simulink model "twoLinkManipulator"  (R2020a)
settings: Solver=ode45  StartTime=0.0  StopTime=20  MaxStep=0.01  RelTol=1e-3
undefined symbols (not defined in the file): DESIRED_TRAJECTORY_IS_FIXED, dq_max, dq_min, k1, k2, k3, q_des_amp, q_des_bias, q_des_freq, q_des_phase, q_max, q_min
libraries: sm_lib x9, nesl_utility x9
settings Model: Creator=bpc  LastModifiedBy=bpc
settings ExplorerConfigSet: InternalSimMechanicsExplorerSettings="<ExplorerConfiguration><canonicalview>aerospace</canonicalview><AnimationSetting><BasePlaybackSpeed>1.0</BasePlaybackSpeed><PlaybackSpeedFactor>1.0</PlaybackSpeedFactor></AnimationSetting><TilePanel><TileInfo><Tiles Columns=\"1\" Count=\"1\" Rows=\"1\"><Column Weight=\"1\"/><Row Weight=\"1\"/><Tile Height=\"1\" Width=\"1\" X=\"0\" Y=\"0\"/></Tiles></TileInfo><SceneInfo><SceneViewer><BGColor><R>0.800000011920928955</R><G>0.800000011920928955</G><B>0.800000011920928955</B></BGColor><Camera><DoPerspective>off</DoPerspective><Position><X>0.880734530182891495</X><Y>-0.069313660265544183</Y><Z>1.00000000000000044</Z></Position><Center><X>0.880734530182891495</X><Y>-0.069313660265544183</Y><Z>4.44089209850062616e-16</Z></Center><Up><X>0</X><Y>1</Y><Z>-0</Z></Up><ViewLimDist>1</ViewLimDist><YLim>0.716863440183610257</YLim><XLim>1.28420727523043032</XLim></Camera></SceneViewer></SceneInfo></TilePanel><MechEditorPanel><Cameras/><GfxPanelCameraMap/><VideoCreator><PlaybackSpeedRatio>1.0</PlaybackSpeedRatio><FrameRate>30</FrameRate><VideoFormat>Motion JPEG AVI</VideoFormat><FrameSize>auto</FrameSize></VideoCreator></MechEditorPanel></ExplorerConfiguration>"

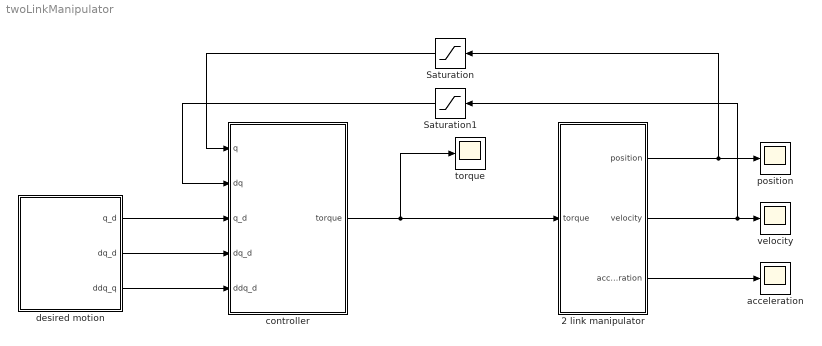
== system twoLinkManipulator ==
  2 link manipulator : Subsystem
  Saturation : Saturate  UpperLimit=q_max-0.001  LowerLimit=q_min+0.001
  Saturation1 : Saturate  UpperLimit=dq_max-0.001  LowerLimit=dq_min+0.001
  acceleration : Scope
  controller : Subsystem
  desired motion : Subsystem
  position : Scope
  torque : Scope
  velocity : Scope
  wires:
  2 link manipulator/1(position) -> Saturation/1, position/1
  2 link manipulator/2(velocity) -> Saturation1/1, velocity/1
  2 link manipulator/3(acceleration) -> acceleration/1
  controller/1(torque) -> 2 link manipulator/1(torque), torque/1
  desired motion/1(q_d) -> controller/3(q_d)
  desired motion/2(dq_d) -> controller/4(dq_d)
  desired motion/3(ddq_q) -> controller/5(ddq_d)
  Saturation/1 -> controller/1(q)
  Saturation1/1 -> controller/2(dq)

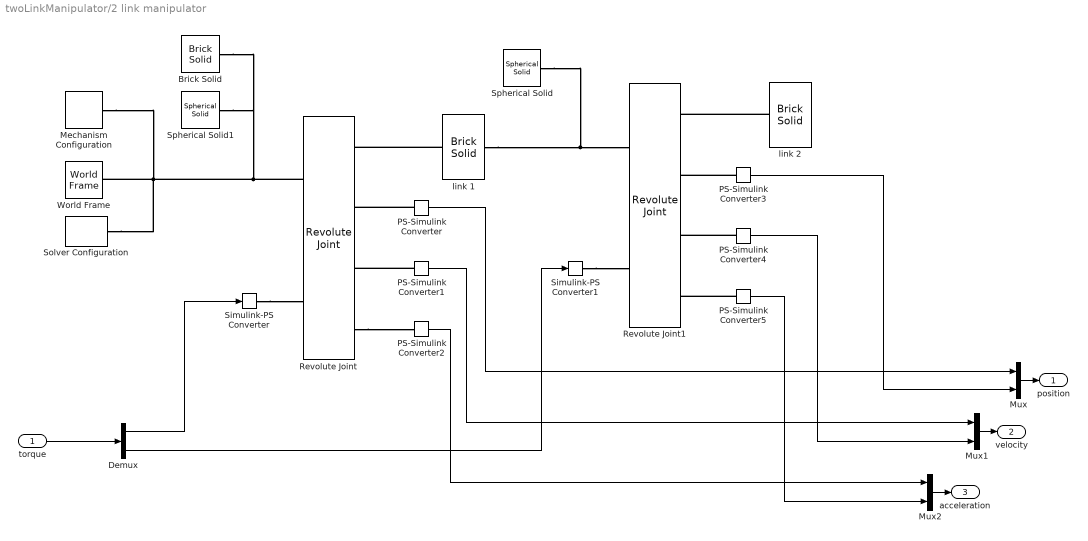
== system twoLinkManipulator/2 link manipulator ==
  torque : Inport
  Brick Solid : sm_lib/Body Elements/Brick Solid  GraphicAmbientColor=[0.15 0.15 0.15 1.0]  BasedOnType=Density  BrickDimensions=[0.2 0.5 0.5]  BrickDimensionUnits=m  CenterOfMass=[0 0 0]  CenterOfMassUnits=m  GraphicDiffuseColor=[0.5 0.5 0.5]  Density=1000  DensityUnits=kg/m^3  DoExposeReferenceFrame=off  GraphicEmissiveColor=[0.0 0.0 0.0 1.0]  ExportEntireGeometry=off  SerializedFrames=<Frames><Frame><Id>Frame1</Id><Value><Name>F1</Name><Origin><Source>GeometricFeature</Source><FeatureName>+x surface</FeatureName></Origin><PrimaryAxis><DefinedDirection>+Z</DefinedDirection><Source>ReferenceFrame</Source><SourceDirection>+Z</SourceDirection><FeatureName></FeatureName></PrimaryAxis><SecondaryAxis><DefinedDirection>+X</DefinedDirection><Source>ReferenceFrame</Source><SourceDirection>+X</SourceDirection><FeatureName></FeatureName></SecondaryAxis></Value></Frame></Frames>  MarkerShape=Sphere  MarkerSize=10  GraphicType=FromGeometry  InertiaType=PointMass  Mass=0.0  MassUnits=kg  MomentsOfInertia=[1 1 1]  MomentsOfInertiaUnits=kg*m^2  GraphicOpacity=1.0  ProductsOfInertia=[0 0 0]  ProductsOfInertiaUnits=kg*m^2  GraphicShininess=75  GraphicSpecularColor=[0.5 0.5 0.5 1.0]  GraphicVisPropType=SimpleVisualProperties
  Demux : Demux  Outputs=2
  Mechanism Configuration : sm_lib/Utilities/Mechanism Configuration  UniformGravity=Constant  GravityVector=[0 -9.80665 0]  GravityUnits=m/s^2  LinearizationDelta=0.001
  Mux : Mux  Inputs=2
  Mux1 : Mux  Inputs=2
  Mux2 : Mux  Inputs=2
  PS-Simulink Converter{,1..5} (6 alike) : nesl_utility/PS-Simulink Converter  PhysicalDomain=network_engine_domain  SubClassName=ps_output  LeftPortType=input  RightPortType=output  PseudoPeriodic=off  Frequencies=[]  Unit=inherit  AffineConversion=off
  Revolute Joint : sm_lib/Joints/Revolute Joint  JointMode=Normal  SenseConstraintForce=off  SenseConstraintForceX=off  SenseConstraintForceY=off  SenseConstraintForceZ=off  SenseConstraintTorque=off  SenseConstraintTorqueX=off  SenseConstraintTorqueY=off  SenseConstraintTorqueZ=off  SenseTotalForce=off  SenseTotalForceX=off  SenseTotalForceY=off  SenseTotalForceZ=off  SenseTotalTorque=off  SenseTotalTorqueX=off  SenseTotalTorqueY=off  SenseTotalTorqueZ=off  CompositeWrenchDir=FollowerOnBase  CompositeWrenchFrame=BaseFrame  EquilibriumPosition=0  EquilibriumPositionUnits=deg  SpringStiffness=0  SpringStiffnessUnits=N*m/deg  DampingCoefficient=0  DampingCoefficientUnits=N*m/(deg/s)  TorqueActuationMode=InputTorque  MotionActuationMode=ComputedMotion  SensePosition=on  SenseVelocity=on  SenseAcceleration=on  SenseTorqueForce=off  SenseLowerLimitTorqueForce=off  SenseUpperLimitTorqueForce=off  LowerLimitSpecify=on  LowerLimitBound=-90  LowerLimitBoundUnits=deg  LowerLimitStiffness=1e4  LowerLimitStiffnessUnits=N*m/deg  LowerLimitDamping=10  LowerLimitDampingUnits=N*m/(deg/s)  LowerLimitTransitionRegionWidth=0.1  LowerLimitTransitionRegionWidthUnits=deg  UpperLimitSpecify=on  UpperLimitBound=90  UpperLimitBoundUnits=deg  UpperLimitStiffness=1e4  UpperLimitStiffnessUnits=N*m/deg  UpperLimitDamping=10  UpperLimitDampingUnits=N*m/(deg/s)  UpperLimitTransitionRegionWidth=0.1  UpperLimitTransitionRegionWidthUnits=deg  PositionTargetSpecify=off  PositionTargetPriority=High  PositionTargetValue=pi/10  PositionTargetValueUnits=rad  VelocityTargetSpecify=off  VelocityTargetPriority=High  VelocityTargetValue=0  VelocityTargetValueUnits=deg/s
  Revolute Joint1 : sm_lib/Joints/Revolute Joint  JointMode=Normal  SenseConstraintForce=off  SenseConstraintForceX=off  SenseConstraintForceY=off  SenseConstraintForceZ=off  SenseConstraintTorque=off  SenseConstraintTorqueX=off  SenseConstraintTorqueY=off  SenseConstraintTorqueZ=off  SenseTotalForce=off  SenseTotalForceX=off  SenseTotalForceY=off  SenseTotalForceZ=off  SenseTotalTorque=off  SenseTotalTorqueX=off  SenseTotalTorqueY=off  SenseTotalTorqueZ=off  CompositeWrenchDir=FollowerOnBase  CompositeWrenchFrame=BaseFrame  EquilibriumPosition=0  EquilibriumPositionUnits=deg  SpringStiffness=0  SpringStiffnessUnits=N*m/deg  DampingCoefficient=0  DampingCoefficientUnits=N*m/(deg/s)  TorqueActuationMode=InputTorque  MotionActuationMode=ComputedMotion  SensePosition=on  SenseVelocity=on  SenseAcceleration=on  SenseTorqueForce=off  SenseLowerLimitTorqueForce=off  SenseUpperLimitTorqueForce=off  LowerLimitSpecify=on  LowerLimitBound=-90  LowerLimitBoundUnits=deg  LowerLimitStiffness=1e4  LowerLimitStiffnessUnits=N*m/deg  LowerLimitDamping=10  LowerLimitDampingUnits=N*m/(deg/s)  LowerLimitTransitionRegionWidth=0.1  LowerLimitTransitionRegionWidthUnits=deg  UpperLimitSpecify=on  UpperLimitBound=90  UpperLimitBoundUnits=deg  UpperLimitStiffness=1e4  UpperLimitStiffnessUnits=N*m/deg  UpperLimitDamping=10  UpperLimitDampingUnits=N*m/(deg/s)  UpperLimitTransitionRegionWidth=0.1  UpperLimitTransitionRegionWidthUnits=deg  PositionTargetSpecify=off  PositionTargetPriority=High  PositionTargetValue=0  PositionTargetValueUnits=deg  VelocityTargetSpecify=off  VelocityTargetPriority=High  VelocityTargetValue=0  VelocityTargetValueUnits=deg/s
  Simulink-PS Converter : nesl_utility/Simulink-PS Converter  PhysicalDomain=network_engine_domain  SubClassName=ps_input  LeftPortType=input  RightPortType=output  PseudoPeriodic=off  Frequencies=[]  NoiseDistribution=none  NoiseParameters=[]  Unit=1  AffineConversion=off  FilteringAndDerivatives=provide  SimscapeFilterOrder=1  InputFilterTimeConstant=0.001  UdotUserProvided=0
  Simulink-PS Converter1 : nesl_utility/Simulink-PS Converter  PhysicalDomain=network_engine_domain  SubClassName=ps_input  LeftPortType=input  RightPortType=output  PseudoPeriodic=off  Frequencies=[]  NoiseDistribution=none  NoiseParameters=[]  Unit=1  AffineConversion=off  FilteringAndDerivatives=provide  SimscapeFilterOrder=1  InputFilterTimeConstant=0.001  UdotUserProvided=0
  Solver Configuration : nesl_utility/Solver Configuration  PhysicalDomain=network_engine_domain  SubClassName=solver  LeftPortType=input  RightPortType=generic  Tones=[]  Harmonics=[]  SimulateNoise=off  Profile=off  UseLocalSampling=off  EnableSwitchedLinearOptims=on  FrequencyDomain=off  UseCCode=off  RelTol=0.001  AbsTol=1e-06  MinStep=1e-09  ToWorkspace=off  RevertToSquareIcSolve=off  NumHomotopyIterations=100  PhasorMode=off  PhasorModeNumHarmonics=1  DoDC=off  ResidualTolerance=1e-09  UseLocalSolver=off  LocalSolverChoice=NE_BACKWARD_EULER_ADVANCER  LocalSolverSampleTime=0.001  DoFixedCost=off  MaxNonlinIter=3  MaxModeIter=2  LinearAlgebra=auto  EquationFormulation=NE_TIME_EF  DelaysMemoryBudget=1024  AutomaticFiltering=on  FilteringTimeConstant=0.001  PartitionStorageMethod=AS_NEEDED  PartitionMemoryBudget=1024  PartitionMethod=ROBUST
  Spherical Solid : sm_lib/Body Elements/Spherical Solid  GraphicAmbientColor=[0.15 0.15 0.15 1.0]  BasedOnType=Density  CenterOfMass=[0 0 0]  CenterOfMassUnits=m  GraphicDiffuseColor=[1.0 0.6 0.2]  Density=1000  DensityUnits=kg/m^3  DoExposeReferenceFrame=on  GraphicEmissiveColor=[0.0 0.0 0.0 1.0]  ExportEntireGeometry=off  SerializedExposedGeometries=<ExposedGeometries/>  SerializedFrames=<Frames/>  MarkerShape=Sphere  MarkerSize=10  GraphicType=FromGeometry  InertiaType=PointMass  Mass=0.0  MassUnits=kg  MomentsOfInertia=[1 1 1]  MomentsOfInertiaUnits=kg*m^2  GraphicOpacity=1.0  ProductsOfInertia=[0 0 0]  ProductsOfInertiaUnits=kg*m^2  GraphicShininess=75  GraphicSpecularColor=[0.5 0.5 0.5 1.0]  SphereRadius=0.02  SphereRadiusUnits=m  GraphicVisPropType=SimpleVisualProperties
  Spherical Solid1 : sm_lib/Body Elements/Spherical Solid  GraphicAmbientColor=[0.15 0.15 0.15 1.0]  BasedOnType=Density  CenterOfMass=[0 0 0]  CenterOfMassUnits=m  GraphicDiffuseColor=[1.0 0.6 0.2]  Density=1000  DensityUnits=kg/m^3  DoExposeReferenceFrame=on  GraphicEmissiveColor=[0.0 0.0 0.0 1.0]  ExportEntireGeometry=off  SerializedExposedGeometries=<ExposedGeometries/>  SerializedFrames=<Frames/>  MarkerShape=Sphere  MarkerSize=10  GraphicType=FromGeometry  InertiaType=PointMass  Mass=0.0  MassUnits=kg  MomentsOfInertia=[1 1 1]  MomentsOfInertiaUnits=kg*m^2  GraphicOpacity=1.0  ProductsOfInertia=[0 0 0]  ProductsOfInertiaUnits=kg*m^2  GraphicShininess=75  GraphicSpecularColor=[0.5 0.5 0.5 1.0]  SphereRadius=0.02  SphereRadiusUnits=m  GraphicVisPropType=SimpleVisualProperties
  World Frame : sm_lib/Frames and Transforms/World Frame
  link 1 : sm_lib/Body Elements/Brick Solid  GraphicAmbientColor=[0.15 0.15 0.15 1.0]  BasedOnType=Density  BrickDimensions=[0.5 0.015 0.015]  BrickDimensionUnits=m  CenterOfMass=[0.25 0.0075 0.0075]  CenterOfMassUnits=m  GraphicDiffuseColor=[0.0 0.0 1.0]  Density=1000  DensityUnits=kg/m^3  DoExposeReferenceFrame=off  GraphicEmissiveColor=[0.0 0.0 0.0 1.0]  ExportEntireGeometry=off  SerializedFrames=<Frames><Frame><Id>Frame1</Id><Value><Name>F1</Name><Origin><Source>GeometricFeature</Source><FeatureName>-x surface</FeatureName></Origin><PrimaryAxis><DefinedDirection>+Z</DefinedDirection><Source>ReferenceFrame</Source><SourceDirection>+Z</SourceDirection><FeatureName></FeatureName></PrimaryAxis><SecondaryAxis><DefinedDirection>+X</DefinedDirection><Source>ReferenceFrame</Source><SourceDirection>+X</SourceDirection><FeatureName></FeatureName></SecondaryAxis></Value></Frame><Frame><Id>Frame2</Id><Value><Name>F2</Name><Origin><Source>GeometricFeature</Source><FeatureName>+x surface</FeatureName></Origin><PrimaryAxis><DefinedDirection>+Z</DefinedDirection><Source>ReferenceFrame</Source><SourceDirection>+Z</SourceDirection><FeatureName></FeatureName></PrimaryAxis><SecondaryAxis><DefinedDirection>+X</DefinedDirection><Source>ReferenceFrame</Source><SourceDirection>+X</SourceDirection><FeatureName></FeatureName></SecondaryAxis></Value></Frame></Frames>  MarkerShape=Sphere  MarkerSize=10  GraphicType=FromGeometry  InertiaType=PointMass  Mass=2  MassUnits=kg  MomentsOfInertia=[0 0.0417 0]  MomentsOfInertiaUnits=kg*m^2  GraphicOpacity=1.0  ProductsOfInertia=[0 0 0]  ProductsOfInertiaUnits=kg*m^2  GraphicShininess=75  GraphicSpecularColor=[0.5 0.5 0.5 1.0]  GraphicVisPropType=SimpleVisualProperties
  link 2 : sm_lib/Body Elements/Brick Solid  GraphicAmbientColor=[0.15 0.15 0.15 1.0]  BasedOnType=Density  BrickDimensions=[0.35 0.015 0.015]  BrickDimensionUnits=m  CenterOfMass=[0.175 0.0075 0.0075]  CenterOfMassUnits=m  GraphicDiffuseColor=[0.0 1.0 0.2]  Density=1000  DensityUnits=kg/m^3  DoExposeReferenceFrame=off  GraphicEmissiveColor=[0.0 0.0 0.0 1.0]  ExportEntireGeometry=off  SerializedFrames=<Frames><Frame><Id>Frame1</Id><Value><Name>F1</Name><Origin><Source>GeometricFeature</Source><FeatureName>-x surface</FeatureName></Origin><PrimaryAxis><DefinedDirection>+Z</DefinedDirection><Source>ReferenceFrame</Source><SourceDirection>+Z</SourceDirection><FeatureName></FeatureName></PrimaryAxis><SecondaryAxis><DefinedDirection>+X</DefinedDirection><Source>ReferenceFrame</Source><SourceDirection>+X</SourceDirection><FeatureName></FeatureName></SecondaryAxis></Value></Frame></Frames>  MarkerShape=Sphere  MarkerSize=10  GraphicType=FromGeometry  InertiaType=PointMass  Mass=1.5  MassUnits=kg  MomentsOfInertia=[0 0.0153 0]  MomentsOfInertiaUnits=kg*m^2  GraphicOpacity=1.0  ProductsOfInertia=[0 0 0]  ProductsOfInertiaUnits=kg*m^2  GraphicShininess=75  GraphicSpecularColor=[0.5 0.5 0.5 1.0]  GraphicVisPropType=SimpleVisualProperties
  position : Outport
  velocity : Outport  Port=2
  acceleration : Outport  Port=3
  wires:
  PS-Simulink Converter/1 -> Mux/1
  PS-Simulink Converter5/1 -> Mux2/2
  PS-Simulink Converter3/1 -> Mux/2
  PS-Simulink Converter4/1 -> Mux1/2
  PS-Simulink Converter1/1 -> Mux1/1
  PS-Simulink Converter2/1 -> Mux2/1
  Mux2/1 -> acceleration/1
  Mux1/1 -> velocity/1
  Mux/1 -> position/1
  torque/1 -> Demux/1
  Demux/1 -> Simulink-PS Converter/1
  Demux/2 -> Simulink-PS Converter1/1
  connections:
  PS-Simulink Converter5/LConn1 -- Revolute Joint1/RConn4
  PS-Simulink Converter4/LConn1 -- Revolute Joint1/RConn3
  link 1/RConn1 -- Spherical Solid/RConn1 -- Revolute Joint1/LConn1
  PS-Simulink Converter3/LConn1 -- Revolute Joint1/RConn2
  Revolute Joint/LConn1 -- Brick Solid/LConn1 -- Spherical Solid1/RConn1 -- Solver Configuration/RConn1 -- Mechanism Configuration/RConn1 -- World Frame/RConn1
  PS-Simulink Converter/LConn1 -- Revolute Joint/RConn2
  link 1/LConn1 -- Revolute Joint/RConn1
  PS-Simulink Converter1/LConn1 -- Revolute Joint/RConn3
  Revolute Joint/RConn4 -- PS-Simulink Converter2/LConn1
  link 2/LConn1 -- Revolute Joint1/RConn1
  Simulink-PS Converter/RConn1 -- Revolute Joint/LConn2
  Simulink-PS Converter1/RConn1 -- Revolute Joint1/LConn2

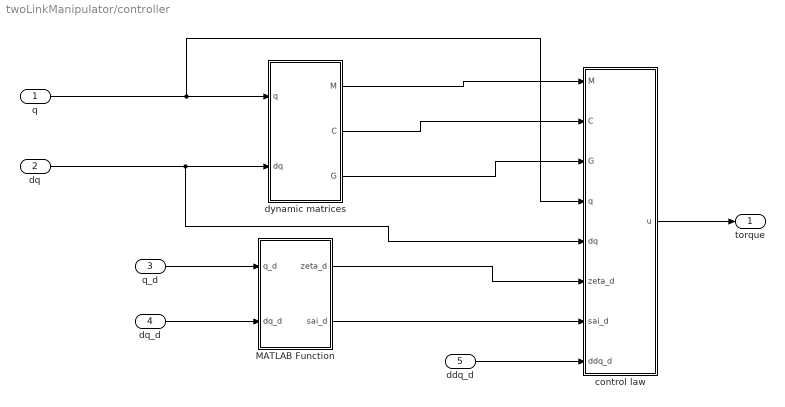
== system twoLinkManipulator/controller ==
  q : Inport
  dq : Inport  Port=2
  q_d : Inport  Port=3
  dq_d : Inport  Port=4
  ddq_d : Inport  Port=5
  MATLAB Function : MATLAB Function  TreatAsAtomicUnit=on
  control law : MATLAB Function  TreatAsAtomicUnit=on
  dynamic matrices : MATLAB Function  TreatAsAtomicUnit=on
  torque : Outport
  wires:
  q/1 -> control law/4(q), dynamic matrices/1(q)
  dq/1 -> control law/5(dq), dynamic matrices/2(dq)
  dynamic matrices/1(M) -> control law/1(M)
  dynamic matrices/2(C) -> control law/2(C)
  dynamic matrices/3(G) -> control law/3(G)
  ddq_d/1 -> control law/8(ddq_d)
  control law/1(u) -> torque/1
  MATLAB Function/1(zeta_d) -> control law/6(zeta_d)
  MATLAB Function/2(sai_d) -> control law/7(sai_d)
  q_d/1 -> MATLAB Function/1(q_d)
  dq_d/1 -> MATLAB Function/2(dq_d)

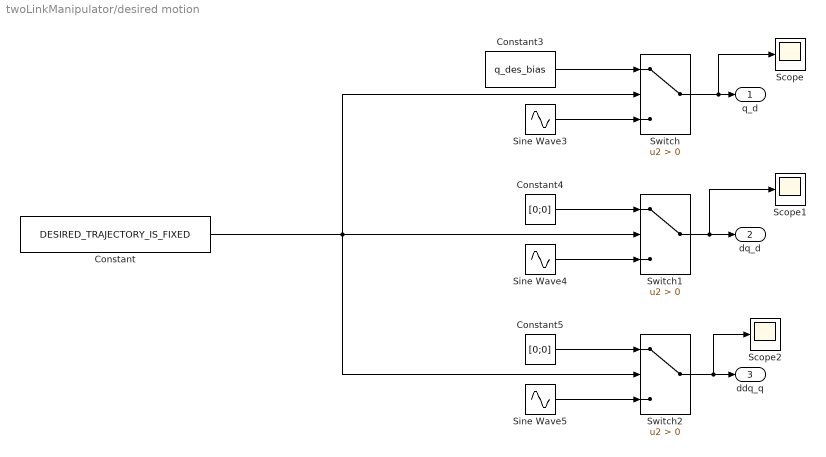
== system twoLinkManipulator/desired motion ==
  Constant : Constant  Value=DESIRED_TRAJECTORY_IS_FIXED
  Constant3 : Constant  Value=q_des_bias
  Constant4 : Constant  Value=[0;0]
  Constant5 : Constant  Value=[0;0]
  Scope : Scope
  Scope1 : Scope
  Scope2 : Scope
  Sine Wave3 : Sin  Amplitude=q_des_amp  Bias=q_des_bias  Frequency=q_des_freq  Phase=q_des_phase  SampleTime=0
  Sine Wave4 : Sin  Amplitude=q_des_amp .* q_des_freq  Bias=[0;0]  Frequency=q_des_freq  Phase=q_des_phase+pi/2  SampleTime=0
  Sine Wave5 : Sin  Amplitude=-q_des_amp .* (q_des_freq .^ 2)  Bias=[0;0]  Frequency=q_des_freq  Phase=q_des_phase  SampleTime=0
  Switch : Switch  Criteria=u2 > Threshold
  Switch1 : Switch  Criteria=u2 > Threshold
  Switch2 : Switch  Criteria=u2 > Threshold
  q_d : Outport
  dq_d : Outport  Port=2
  ddq_q : Outport  Port=3
  wires:
  Switch/1 -> Scope/1, q_d/1
  Switch1/1 -> Scope1/1, dq_d/1
  Switch2/1 -> Scope2/1, ddq_q/1
  Constant/1 -> Switch1/2, Switch2/2, Switch/2
  Constant3/1 -> Switch/1
  Sine Wave3/1 -> Switch/3
  Sine Wave4/1 -> Switch1/3
  Constant4/1 -> Switch1/1
  Constant5/1 -> Switch2/1
  Sine Wave5/1 -> Switch2/3

== matlab function twoLinkManipulator/controller/control law ==
  data: M input; C input; G input; q input; u output; dq input; zeta_d input; sai_d input; ddq_d input; q_min parameter; q_max parameter; dq_min parameter; dq_max parameter; k1 parameter; k2 parameter; k3 parameter
function u = fcn(M,C,G,q,dq,zeta_d,sai_d,ddq_d, q_min, q_max, dq_min, dq_max, k1, k2, k3)

%%%%%%%%%%%%%%%%%%%%%%%%%%%%%%%%%%%%%%%%%%%%%%%%%%%%%%%%%%%%%%%%%%%%%%%%%

q_avg = (q_max+q_min)/2;
dq_avg = (dq_max+dq_min)/2;

delta_q = diag((q_max-q_min)/2);
delta_dq = diag((dq_max-dq_min)/2);

%%%%%%%%%%%%%%%%%%%%%%%%%%%%%%%%%%%%%%%%%%%%%%%%%%%%%%%%%%%%%%%%%%%%%%%%%

zeta = atanh(delta_q\(q-q_avg));
sai = atanh(delta_dq\(dq-dq_avg));

%%%%%%%%%%%%%%%%%%%%%%%%%%%%%%%%%%%%%%%%%%%%%%%%%%%%%%%%%%%%%%%%%%%%%%%%%

J_zeta = delta_q*(eye(2)-diag(tanh(zeta))^2);
J_zeta_d = delta_q*(eye(2)-diag(tanh(zeta_d))^2);

J_sai = delta_dq*(eye(2)-diag(tanh(sai))^2);
J_sai_d = delta_dq*(eye(2)-diag(tanh(sai_d))^2);

%%%%%%%%%%%%%%%%%%%%%%%%%%%%%%%%%%%%%%%%%%%%%%%%%%%%%%%%%%%%%%%%%%%%%%%%%

dzeta = J_zeta\(dq_avg + delta_dq*tanh(sai));
dzeta_d = J_zeta_d\(dq_avg + delta_dq*tanh(sai_d));

dJ_zeta = -2*diag(tanh(zeta))*J_zeta*diag(dzeta);
dJ_zeta_d = -2*diag(tanh(zeta_d))*J_zeta_d*diag(dzeta_d);

dsai_d = J_sai_d\ddq_d;

%%%%%%%%%%%%%%%%%%%%%%%%%%%%%%%%%%%%%%%%%%%%%%%%%%%%%%%%%%%%%%%%%%%%%%%%%

p = 15;

tanh_bsai_r = delta_dq\(J_zeta/J_zeta_d*(dq_avg+delta_dq*tanh(sai_d)) - dq_avg);
sai_r =  atanh(tanh_bsai_r./(1+abs(tanh_bsai_r).^p).^(1/p));

J_sai_r = delta_dq*(eye(2)-diag(tanh(sai_r))^2);

dsai_r = J_sai_r\(dJ_zeta/J_zeta_d*(dq_avg+delta_dq*tanh(sai_d)) ...
    -J_zeta/J_zeta_d*dJ_zeta_d/J_zeta_d*(dq_avg+delta_dq*tanh(sai_d)) ...
    +J_zeta/J_zeta_d*delta_dq*(eye(2)-diag(tanh(sai_d))^2)*dsai_d);

%%%%%%%%%%%%%%%%%%%%%%%%%%%%%%%%%%%%%%%%%%%%%%%%%%%%%%%%%%%%%%%%%%%%%%%%%

e_zeta = zeta-zeta_d;
e_sai = sai-sai_r;

%%%%%%%%%%%%%%%%%%%%%%%%%%%%%%%%%%%%%%%%%%%%%%%%%%%%%%%%%%%%%%%%%%%%%%%%%

u = G + C*dq + M*J_sai*(dsai_r - k2\k1/J_zeta*delta_dq ...
    *(tanh(sai)-tanh(sai_r)) - k2*e_zeta - k3/J_sai*e_sai);

== matlab function twoLinkManipulator/controller/dynamic matrices ==
  data: q input; M output; dq input; C output; G output
function [M,C,G] = fcn(q,dq)

g = 9.81;

m1 = 2;
m2 = 1.5;
l1 = 0.5;
l2 = 0.35;

lc1 = 0.5*l1;
lc2 = 0.5*l2;

I1 = m1*l1^2/12;
I2 = m2*l2^2/12;

%%%%%%%%%%%%%%%%%%%%%%%%%%%%%%%%%%%%%%%%%%%%%%%%%%%%%%%%%%%%%%%%%%%%%%

q1 = q(1);
q2 = q(2);

dq1 = dq(1);
dq2 = dq(2);

M = [ m1*lc1^2 + m2*(l1^2+lc2^2+l1*l2*cos(q2)) + I1 + I2,   m2*(lc2^2+l1*lc2*cos(q2)) + I2
      m2*(lc2^2+l1*lc2*cos(q2)) + I2,                       m2*lc2^2+I2];
  
C = [ -m2*l1*lc2*sin(q2)*dq2,       -m2*l1*lc2*sin(q2)*(dq1+dq2)
       m2*l2*lc2*sin(q2)*dq1,         0];
   
G = [ (m1*lc1+m2*l1)*g*cos(q1) + m2*lc2*g*cos(q1+q2);
       m2*lc2*g*cos(q1+q2)];

== matlab function twoLinkManipulator/controller/MATLAB Function ==
  data: q_d input; zeta_d output; dq_d input; sai_d output; q_min parameter; q_max parameter; dq_min parameter; dq_max parameter
function [zeta_d,sai_d] = fcn(q_d,dq_d, q_min, q_max, dq_min, dq_max)

q_avg = (q_max+q_min)/2;
dq_avg = (dq_max+dq_min)/2;

delta_q = diag((q_max-q_min)/2);
delta_dq = diag((dq_max-dq_min)/2);

%%%%%%%%%%%%%%%%%%%%%%%%%%%%%%%%%%%%%%%%%%%%%%%%%%%%%%%%%%%%%%%%%%%%%%%%%

zeta_d = atanh(delta_q\(q_d-q_avg));
sai_d = atanh(delta_dq\(dq_d-dq_avg));
